simulink model "V_over_F_Control_of_Induction_Motors"  (R2025a)
settings: Solver=ode23tb  StartTime=0.0  StopTime=10  MaxStep=1e-4  RelTol=1e-3
libraries: spsControlledVoltageSourceLib x3, simulink x2, spsAsynchronousMachineSIUnitsLib x1, spspowerguiLib x1
settings Model: Creator=Jawad  LastModifiedBy=Jawad

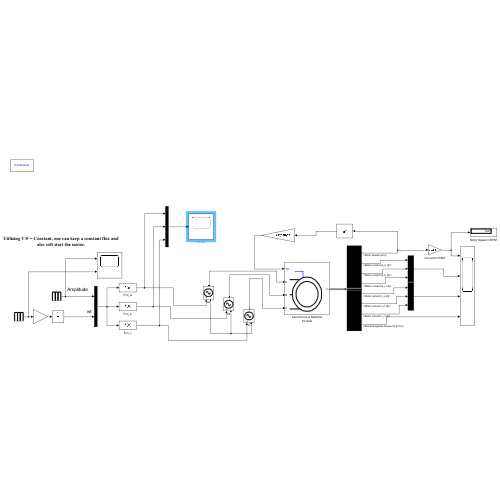
[thumbnail: Simulink's stored preview of the top-level diagram]
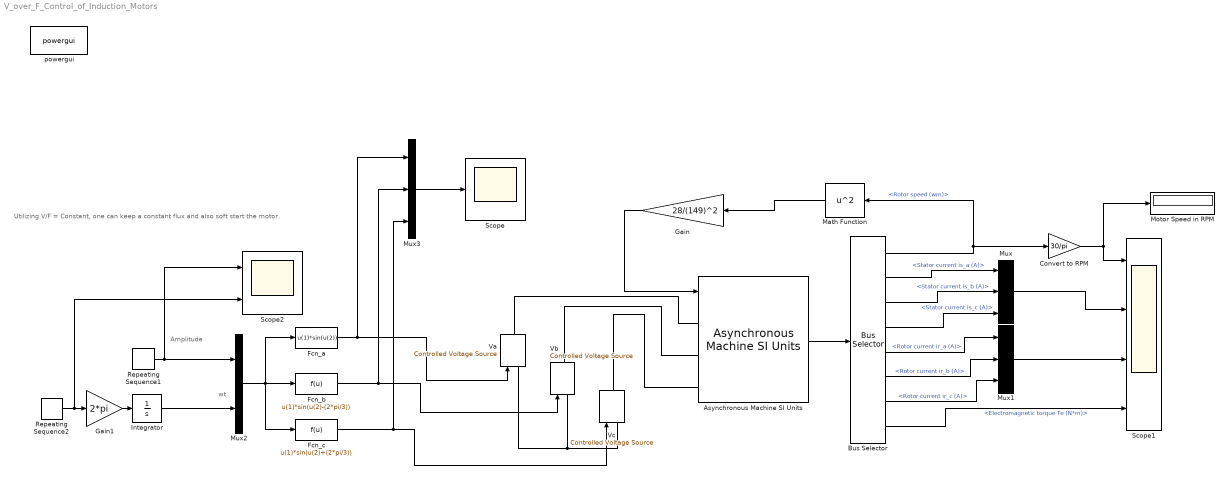
== system V_over_F_Control_of_Induction_Motors ==
  note: Utilizing V/F = Constant, one can keep a constant flux and also soft start the motor.
  note: Amplitude
  note: wt
  Asynchronous Machine SI Units : spsAsynchronousMachineSIUnitsLib/Asynchronous Machine SI Units  RotorType=Squirrel-cage  PresetModel="15:  5.4 HP (4KW)   400 V  50Hz 1430 RPM"  MechanicalLoad=Torque Tm  ShowDetailedParameters=on  ReferenceFrame=Rotor  Units=SI  MeasurementBus=off  NominalParameters=[4000 400 50]  VoltageRatio=1  Stator=[1.405 0.005839]  Rotor=[1.395 0.005839]  Cage1=[0.4155 0.002066]  Cage2=[0.4168 0.0003495]  Lm=0.1722  Mechanical=[0.0131 0.002985 2]  PolePairs=2  InitialConditions=[1 0 0 0 0 0 0 0]  SimulateSaturation=off  Saturation=[14.03593122, 27.81365428, 53.79336849, 72.68890987, 97.98006896, 148.6815601, 215.7428561, 302.9841135, 428.7778367 ; 230, 322, 414, 460, 506, 552, 598, 644, 690]  LoadFlowParameters=1492000  TsPowergui=0  TsBlock=-1  IterativeModel=Trapezoidal non iterative  IterativeDiscreteModel=Trapezoidal non iterative  Pmec=1.492e+006
  Bus Selector : BusSelector  OutputSignals=Mechanical.Rotor speed (wm),Stator measurements.Stator current is_a (A),Stator measurements.Stator current is_b (A),Stator measurements.Stator current is_c (A),Rotor measurements.Rotor current ir_a (A),Rotor measurements.Rotor current ir_b (A),Rotor measurements.Rotor current ir_c (A),Mechanical.Electromagnetic torque Te (N*m)
  Convert to RPM : Gain  Gain=30/pi
  Fcn_a : Fcn  Expr=u(1)*sin(u(2))
  Fcn_b : Fcn  Expr=u(1)*sin(u(2)-(2*pi/3))
  Fcn_c : Fcn  Expr=u(1)*sin(u(2)+(2*pi/3))
  Gain : Gain  Gain=28/(149)^2
  Gain1 : Gain  Gain=2*pi
  Integrator : Integrator
  Math Function : Math  Operator=square
  Motor Speed in RPM : Display
  Mux : Mux  Inputs=3
  Mux1 : Mux  Inputs=3
  Mux2 : Mux  Inputs=2
  Mux3 : Mux  Inputs=3
  Repeating Sequence1 : simulink/Sources/Repeating Sequence  rep_seq_t=[0 0.2 10]  rep_seq_y=[0 327 327]
  Repeating Sequence2 : simulink/Sources/Repeating Sequence  rep_seq_t=[0 0.2 10]  rep_seq_y=[0 50 50]
  Scope : Scope
      settings: ActiveDisplayYMinimum=-408.74700271994726  ActiveDisplayYMaximum=408.74700271995397
  Scope1 : Scope  NumInputPorts=4
      settings: ActiveDisplayString=4  Title=Electromagnetic Torque  ActiveDisplayYMinimum=-15.652982258882908  ActiveDisplayYMaximum=58.898757141380266
  Scope2 : Scope  NumInputPorts=2
      settings: ActiveDisplayYMinimum=-40.874999999999993  ActiveDisplayYMaximum=367.875  DataLoggingVariableName=ScopeData2
  Va : spsControlledVoltageSourceLib/Controlled Voltage Source  Initialize=on  Source_Type=AC  Amplitude=0  Phase=0  Frequency=0  Measurements=None
  Vb : spsControlledVoltageSourceLib/Controlled Voltage Source  Initialize=on  Source_Type=AC  Amplitude=0  Phase=0  Frequency=0  Measurements=None
  Vc : spsControlledVoltageSourceLib/Controlled Voltage Source  Initialize=on  Source_Type=AC  Amplitude=0  Phase=0  Frequency=0  Measurements=None
  powergui : spspowerguiLib/powergui  Priority=1  SimulationMode=Continuous  SampleTime=50e-6  frequency=60  Iterations=50  frequencyindice=50  Pbase=100e6  ErrMax=1e-4  UnitsV=kV  UnitsW=MW  buscounter=0  FunctionMessages=off  echomessages=off  EnableUseOfTLC=off  CurrentSourceSwitches=off  DisableSnubberDevices=off  DisableRonSwitches=off  DisableVfSwitches=off  DisplayEquations=off  AutomaticDiscreteSolvers=off  SolverType=Tustin/Backward Euler (TBE)  Interpol=off  ExternalGateDelay=off  methode=off  Ts=100  x0status=blocks  SPID=on  SwTol=0  HookPort=off  NonlinearTolerance=1e-4  nMaxIteration=100  ContinueOnMaxIteration=off  RestoreLinks=warning  ResistiveCurrentMeasurement=off  Frange=[0:2:500]  Ylog=off  Xlog=on  ShowGrid=off  save=off  variable=ZData  structure=0  ZoomFFT=off  StartTime=0.0  cycles=1  DisplayStyle=1  fundamental=60  FreqAxis=off  MaxFrequency=1000  frequencyindicesteady=1  RmsSteady=1  display=off
  wires:
  Bus Selector/8 -> Scope1/4  "<Electromagnetic torque Te (N*m)>"
  Bus Selector/3 -> Mux/2  "<Stator current is_b (A)>"
  Bus Selector/7 -> Mux1/3  "<Rotor current ir_c (A)>"
  Bus Selector/4 -> Mux/3  "<Stator current is_c (A)>"
  Asynchronous Machine SI Units/1 -> Bus Selector/1
  Bus Selector/1 -> Math Function/1, Convert to RPM/1  "<Rotor speed (wm)>"
  Bus Selector/6 -> Mux1/2  "<Rotor current ir_b (A)>"
  Convert to RPM/1 -> Scope1/1, Motor Speed in RPM/1
  Mux/1 -> Scope1/2
  Bus Selector/2 -> Mux/1  "<Stator current is_a (A)>"
  Math Function/1 -> Gain/1
  Mux1/1 -> Scope1/3
  Bus Selector/5 -> Mux1/1  "<Rotor current ir_a (A)>"
  Gain/1 -> Asynchronous Machine SI Units/1
  Mux2/1 -> Fcn_c/1, Fcn_b/1, Fcn_a/1
  Fcn_b/1 -> Mux3/2, Vb/1
  Fcn_c/1 -> Mux3/3, Vc/1
  Repeating Sequence1/1 -> Scope2/1, Mux2/1
  Repeating Sequence2/1 -> Scope2/2, Gain1/1
  Gain1/1 -> Integrator/1
  Integrator/1 -> Mux2/2
  Mux3/1 -> Scope/1
  Fcn_a/1 -> Mux3/1, Va/1
  connections:
  Vc/LConn1 -- Vb/LConn1 -- Va/LConn1
  Va/RConn1 -- Asynchronous Machine SI Units/LConn1
  Vb/RConn1 -- Asynchronous Machine SI Units/LConn2
  Vc/RConn1 -- Asynchronous Machine SI Units/LConn3
